simulink model "PD_traj"  (R2019b)
settings: Solver=ode23t  StartTime=0.0  StopTime=50  RelTol=1e-3  AbsTol=1e-6
undefined symbols (not defined in the file): a0, a1, a2, a3, dq0, Kd_endEff, Kp_endEff, L_d, parameter, q0, x_endEff_D
libraries: simulink x1
settings Model: Creator=giga4  LastModifiedBy=ariannagasparri
settings SolverCC: AutoScaleAbsTol=off
settings DebuggingCC: SignalRangeChecking=warning
settings SFSimCC: CustomCodeUndefinedFunction=UseInterfaceOnly

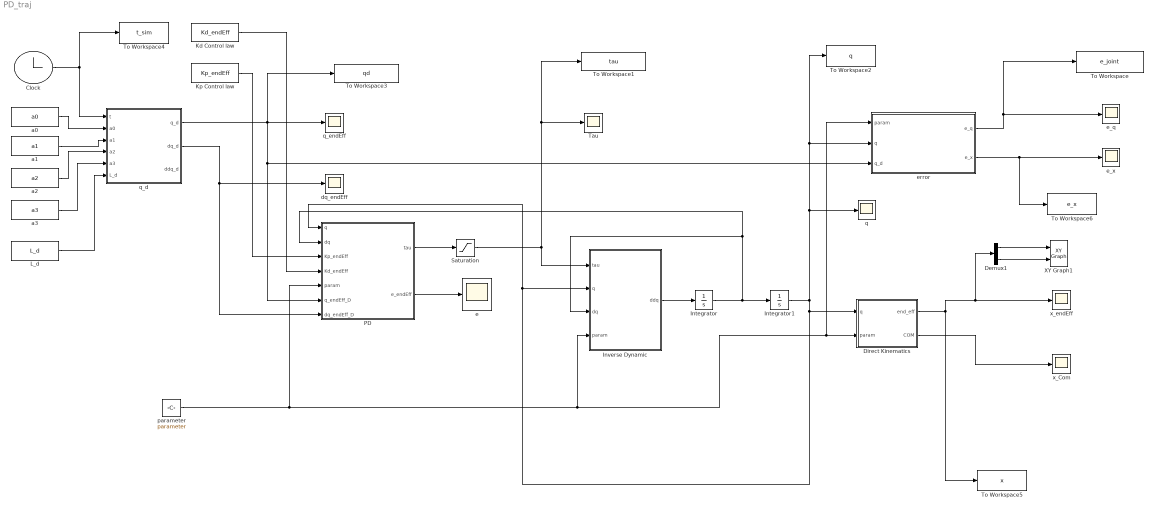
== system PD_traj ==
  Clock : Clock
  Demux1 : Demux  Outputs=3
  "Direct Kinematics " : MATLAB Function  TreatAsAtomicUnit=on
  Integrator : Integrator  InitialCondition=dq0
  Integrator1 : Integrator  InitialCondition=q0
  "Inverse Dynamic " : MATLAB Function  TreatAsAtomicUnit=on
  Kd Control law : Constant  Value=Kd_endEff
  Kp Control law : Constant  Value=Kp_endEff
  L_d : Constant  Value=L_d
  PD : MATLAB Function  TreatAsAtomicUnit=on
  Saturation : Saturate  UpperLimit=800  LowerLimit=-800
  Tau : Scope
  To Workspace : ToWorkspace  VariableName=e_joint  SaveFormat=Structure With Time  SampleTime=-1
      settings: Save2DSignal=2-D array (concatenate along first dimension)
  To Workspace1 : ToWorkspace  VariableName=tau  SaveFormat=Structure With Time  SampleTime=-1
  To Workspace2 : ToWorkspace  VariableName=q  SaveFormat=Structure With Time  SampleTime=-1
  To Workspace3 : ToWorkspace  VariableName=qd  SaveFormat=Structure With Time  SampleTime=-1
  To Workspace4 : ToWorkspace  VariableName=t_sim  SaveFormat=Structure With Time  SampleTime=-1
  To Workspace5 : ToWorkspace  VariableName=x  SaveFormat=Structure With Time  SampleTime=-1
  To Workspace6 : ToWorkspace  VariableName=e_x  SaveFormat=Structure With Time  SampleTime=-1
  XY Graph1 : simulink/Sinks/XY Graph  xmin=x_endEff_D(1)-2  xmax=x_endEff_D(1)+2  ymin=x_endEff_D(3)-2  ymax=x_endEff_D(3)+2  st=-1
  a0 : Constant  Value=a0
  a1 : Constant  Value=a1
  a2 : Constant  Value=a2
  a3 : Constant  Value=a3
  dq_endEff : Scope
  e : Scope
  e_q : Scope
  e_x : Scope
  error : MATLAB Function  TreatAsAtomicUnit=on
  "parameter " : Constant  Value=parameter
  q : Scope
  q_d : MATLAB Function  TreatAsAtomicUnit=on
  q_endEff : Scope
  x_Com : Scope
  x_endEff : Scope
  wires:
  "parameter "/1 -> error/1(param), "Direct Kinematics "/2(param), "Inverse Dynamic "/4(param), PD/5(param)
  "Inverse Dynamic "/1(ddq) -> Integrator/1
  Integrator/1 -> "Inverse Dynamic "/3(dq), PD/2(dq), Integrator1/1
  PD/1(tau) -> Saturation/1
  "Direct Kinematics "/2(COM) -> x_Com/1
  Kp Control law/1 -> PD/3(Kp_endEff)
  Demux1/1 -> XY Graph1/1
  Demux1/3 -> XY Graph1/2
  Clock/1 -> q_d/1(t), To Workspace4/1
  a0/1 -> q_d/2(a0)
  a1/1 -> q_d/3(a1)
  a2/1 -> q_d/4(a2)
  a3/1 -> q_d/5(a3)
  q_d/2(dq_d) -> dq_endEff/1, PD/7(dq_endEff_D)
  q_d/1(q_d) -> error/3(q_d), PD/6(q_endEff_D), To Workspace3/1, q_endEff/1
  Integrator1/1 -> "Direct Kinematics "/1(q), "Inverse Dynamic "/2(q), PD/1(q), To Workspace2/1, error/2(q), q/1
  "Direct Kinematics "/1(end_eff) -> Demux1/1, x_endEff/1, To Workspace5/1
  error/2(e_x) -> To Workspace6/1, e_x/1
  error/1(e_q) -> To Workspace/1, e_q/1
  PD/2(e_endEff) -> e/1
  L_d/1 -> q_d/6(L_d)
  Kd Control law/1 -> PD/4(Kd_endEff)
  Saturation/1 -> Tau/1, To Workspace1/1, "Inverse Dynamic "/1(tau)

== matlab function PD_traj/Direct Kinematics  ==
  data: q input; end_eff output; param input; COM output
function [end_eff, COM] = DirectK(q,param)

    [Pcom, Etip, ~, ~, ~, ~, ~, ~, ~] =  forwardKinematics(param, q);
    
    end_eff = Etip(1:3, 4);
    COM = Pcom;
    
end

== matlab function PD_traj/Inverse Dynamic  ==
  data: tau input size=[6,1]; q input size=[6,1]; dq input size=[6,1]; ddq output size=[6,1]; param input
function ddq = inverseDynamic(tau, q, dq, param)

%     B = B_f(q, param);
%     C = C_f(q, dq, param);
%     G = G_f(q, param);

    B = B_fun(param, q);
    C = C_fun(param, q, dq);
    G = G_fun(param, q);

    ddq = B\(tau - G - C*dq);

end

== matlab function PD_traj/PD ==
  data: q input size=[6,1]; dq input size=[6,1]; Kp_endEff input; Kd_endEff input; tau output; param input; q_endEff_D input size=[6,1]; dq_endEff_D input size=[6,1]; e_endEff output size=[6,1]
function [tau, e_endEff]  = x_now(q, dq, Kp_endEff, Kd_endEff, param, q_endEff_D, dq_endEff_D)

%     B = B_f(q, param);
%     C = C_f(q, dq, param);
%     G = G_f(q, param);

    G = G_fun(param, q);

%     Kp_endEff = K_endEff(1:6,1:6);
%     Kd_endEff = K_endEff(1:6,7:12);
    
    %% controllo Diretto
    e_endEff = q_endEff_D - q;
    de_endEff = dq_endEff_D - dq;
    
    tau = Kp_endEff*e_endEff + Kd_endEff*de_endEff + G;
    
end

== matlab function PD_traj/error ==
  data: param input; q input; e_q output; q_d input; e_x output
function [e_q, e_x]  = error(param, q, q_d)
    

    [~, Etip, ~, ~, ~, ~, ~, ~, ~] =  forwardKinematics(param, q);
    [~, Etip_d, ~, ~, ~, ~, ~, ~, ~] =  forwardKinematics(param, q_d);  

    e_x = Etip_d(1:3,4) - Etip(1:3,4);

    e_q = q_d - q;
    
end

== matlab function PD_traj/q_d ==
  data: t input; q_d output; dq_d output; ddq_d output; a0 input; a1 input; a2 input; a3 input; L_d input
function [q_d, dq_d, ddq_d] = desiderable_q(t, a0, a1, a2, a3, L_d)

    [q_d, dq_d, ddq_d] = vettoreq(a0, a1, a2, a3, t);
end
